simulink model "Model2_V032_R_T4"  (R2023a)
settings: Solver=ode14x  StartTime=0.0  StopTime=Inf  FixedStep=ts  MaxStep=ts  RelTol=1e-5
values from neighbouring files (symbols this model uses):
  ausrollen_a_v = parameters.ausrollen_a_v    [efficiencycalc.m]    (also in parameters_initials.mat = 1)
  bremspunkte = parameters.bremspunkte    [efficiencycalc.m]    (also in parameters_initials.mat = [6100  280  8; 10400  500  3; 14100  550  8; 17729  0  1])
  brennstoffzellen_eta_kennfeld = parameters.brennstoffzellen_eta_kennfeld    [efficiencycalc.m]    (also in parameters_initials.mat = )
  brennstoffzellen_ui_kennfeld = parameters.brennstoffzellen_ui_kennfeld    [efficiencycalc.m]    (also in parameters_initials.mat = )
  coeffs_motor_moment = parameters.coeffs_motor_moment    [efficiencycalc.m]    (also in parameters_initials.mat = [30 30 30 5 7.5 10 0 0 0 6000 6000 6000 ... (30 elements, 3x)
  coeffs_motor_wirkungsgrad = parameters.coeffs_motor_wirkungsgrad    [efficiencycalc.m]    (also in parameters_initials.mat = [30 30 30 5 7.5 10 0 0 0 6000 6000 6000 ... (39 elements, 3x)
  fahrzeug_parameter = parameters.fahrzeug_parameter    [efficiencycalc.m]    (also in parameters_initials.mat = )
  strategie_parameter = parameters.strategie_parameter    [efficiencycalc.m]    (also in parameters_initials.mat = )
  strecke = parameters.strecke    [efficiencycalc.m]    (also in parameters_initials.mat = )
  ts = parameters.ts    [efficiencycalc.m]    (also in parameters_initials.mat = 0.01)
  U_moment = parameters.U_moment    [efficiencycalc.m]    (also in parameters_initials.mat = [30 3])
  U_wirkungsgrad = parameters.U_wirkungsgrad    [efficiencycalc.m]    (also in parameters_initials.mat = [30 3])
  umwelt_parameter = parameters.umwelt_parameter    [efficiencycalc.m]    (also in parameters_initials.mat = )
  zwangsgas = zeros(length(strecke.x),strecke.Rundenzahl)    [Automatisierung_Model_2.m]    (also in efficiencycalc.m; parameters_initials.mat = [0 0 0 0 0 0 0 0 0 0 0 0 ... (2563 elements, 233x11)])
libraries: simulink x1
(part 3 of 3)

== matlab function Model2_V032_R_T4/Motorsteuerung/Kennfeld MC und Motor zusammen/Bestimmung_Wirkungsgrad_aus_Polynomen ==
  data: I input; eta_motor output; U_SC input; n_motor input; eta_U_down output; eta_U_up output; U_wirkungsgrad input; coeffs_motor_wirkungsgrad input; eta_U_down_I_down output; eta_U_down_I_up output; eta_U_up_I_down output; eta_U_up_I_up output
function [eta_motor , eta_U_down , eta_U_up , eta_U_down_I_down , eta_U_down_I_up , eta_U_up_I_down , eta_U_up_I_up ]  = fcn( I , U_SC , n_motor , U_wirkungsgrad , coeffs_motor_wirkungsgrad )
%% Bestimmung Wirkungsgrad aus Polynomen
% Hydro2Motion
% Prototyp: Homer
% Stand: 23.01.2020
% edited: Robin Nedella

%% Eingang
% I:                        [A]     aktuell gefahrener Strom
% U_SC:                     [V]     aktuelle Spannung in den SuperCaps, also aktuelle Spannung am Motorcontroller
% n_motor:                  [rps]   aktuelle Motordrehzahl
% coeffs_motor_wirkungsgrad:[]      Matrix, in welcher die Koeffizienten der Polynome hinterlegt sind (Spalte 1: Strom, 2: Spanung, ab 3: Koeffizienten)
% U_wirkungsgrad:           [V]     Vektor, in welchem die Spannungen stehen, welche in coeffs hinterlegt

%% Ausgang
% eta_motor:                [-]     aktueller Wirkungsgrad Motor bei aktuellem Strom und aktueller Spannung
% eta_U_down:               [-]     aktueller Wirkungsgrad Motor bei nächst kleinerem Strom und aktueller Spannung
% eta_U_up:                 [-]     aktueller Wirkungsgrad Motor bei nächst größerem Strom und aktueller Spannung

%%
n_motor = n_motor * 60; % Polynome basieren auf RPM, nicht RPS

%% Initialisierung
U_down = 0; % nächst kleinere Spannung, für welche Polynome hinterlegt
U_up = 0;   % nächst größere Spannung, für welche Polynome hinterlegt

U_down_I_down = 0; % nächst kleinerer Strom für untere Spannung, für welchen Polynom hinterlegt
U_up_I_down = 0;   % nächst kleinerer Strom für obere Spannung, für welchen Polynom hinterlegt
U_down_I_up = 0;   % nächst größerer Strom für untere Spannung, für welchen Polynom hinterlegt
U_up_I_up = 0;     % nächst größerer Strom für obere Spannung, für welchen Polynom hinterlegt

I_U_down = zeros(1,2);
I_U_up = zeros(1,2);

row_U_down_I_down = 0;  % Zeile, in welcher Koeffizienten für nächst kleineren Strom und nächst kleineren Spannung steht
row_U_down_I_up = 0;    % Zeile, in welcher Koeffizienten für nächst kleineren Strom und nächst größeren Spannung steht
row_U_up_I_down = 0;    % Zeile, in welcher Koeffizienten für nächst größeren Strom und nächst kleineren Spannung steht
row_U_up_I_up = 0;      % Zeile, in welcher Koeffizienten für nächst größeren Strom und nächst größerer Spannung steht

n_motor_U_down_I_down = 0;  % Motordrehzahl, mit welcher das Polynom ausgewertet wird (Gültigkeitsbereich Polynom beachtet) nächst kleinere Spannung und nächst kleinerer Strom
n_motor_U_down_I_up = 0;    % Motordrehzahl, mit welcher das Polynom ausgewertet wird (Gültigkeitsbereich Polynom beachtet) nächst kleinere Spannung und nächst größerer Strom
n_motor_U_up_I_down = 0;    % Motordrehzahl, mit welcher das Polynom ausgewertet wird (Gültigkeitsbereich Polynom beachtet) nächst größere Spannung und nächst kleinerer Strom
n_motor_U_up_I_up = 0;      % Motordrehzahl, mit welcher das Polynom ausgewertet wird (Gültigkeitsbereich Polynom beachtet) nächst größere Spannung und nächst größerer Strom

eta_U_down_I_down = 0;  % aktueller Wirkungsgrad bei nächst kleinerer Spannung und nächst kleinerem Strom
eta_U_down_I_up = 0;    % aktueller Wirkungsgrad bei nächst kleinerer Spannung und nächst größerem Strom
eta_U_up_I_down = 0;    % aktueller Wirkungsgrad bei nächst größerer Spannung und nächst kleinerem Strom
eta_U_up_I_up = 0;      % aktueller Wirkungsgrad bei nächst größerer Spannung und nächst größerem Strom

eta_U_down = 0;         % aktueller Wirkungsgrad bei nächst kleinerer Spannung und aktuellem Strom
eta_U_up = 0;           % aktueller Wirkungsgrad bei nächst größerer Spannung und aktuellem Strom

eta_motor = 1;          % aktueller Wirkungsgrad bei aktuellem Strom und aktueller Spannung (hier: Initialisierung)
%%
if I ~= 0   % wenn gleich null, dann eta_motor = 0 (es muss nichts berechnet werden)
    
    %% suche 2 nächsten Spannungen
        % wenn unter kleinster: nimm kleinste Spannung
    if U_SC < U_wirkungsgrad(1,1)       % wenn aktuelle Spannung kleiner als kleinste im KF hinterlegte
        U_down = U_wirkungsgrad(1,1);       % nächst kleinere Spannung ist kleinste hinterlegte Spannung
        U_up = U_wirkungsgrad(1,1);         % nächst größere Spannung ist kleinste hinterlegte Spannung
        I_U_down = zeros(U_wirkungsgrad(1,2),2);       % Initialisierung des Vektors, wo Ströme, welche bei nächst kleinerer Spannung im Kennfeld hinterlegt sind, gespeichert werden
        I_U_up = zeros(U_wirkungsgrad(1,2),2);         % Initialisierung des Vektors, wo Ströme, welche bei nächst größerer Spannung im Kennfeld hinterlegt sind, gespeichert werden
    elseif U_SC > U_wirkungsgrad(end,1) % wenn aktuelle Spannung größer als größte im KF hinterlegte
        U_down = U_wirkungsgrad(end,1);     % nächst kleinere Spannung ist größte hinterlegte Spannung
        U_up = U_wirkungsgrad(end,1);       % nächst größere Spannung ist größte hinterlegte Spannung
        I_U_down = zeros(U_wirkungsgrad(end,2),2);       % Initialisierung des Vektors, wo Ströme, welche bei nächst kleinerer Spannung im Kennfeld hinterlegt sind, gespeichert werden
        I_U_up = zeros(U_wirkungsgrad(end,2),2);         % Initialisierung des Vektors, wo Ströme, welche bei nächst größerer Spannung im Kennfeld hinterlegt sind, gespeichert werden
    else                                % dann liegt aktuelle Spannung an den Grenzen der m KF hinterlegten Spannungen oder dazwischen
        for j = 1:1:length(U_wirkungsgrad)  % prüfe, ob die gefahrene Spannung direkt im KF hinterlegt ist
           if U_SC == U_wirkungsgrad(j)         % wenn die gefahrene Spannung direkt im KF hinterlegt ist
               U_down = U_SC;                       % dann muss nicht interpoliert werden
               U_up = U_SC;
               I_U_down = zeros(U_wirkungsgrad(j,2),2);       % Initialisierung des Vektors, wo Ströme, welche bei nächst kleinerer Spannung im Kennfeld hinterlegt sind, gespeichert werden
               I_U_up = zeros(U_wirkungsgrad(j,2),2);         % Initialisierung des Vektors, wo Ströme, welche bei nächst größerer Spannung im Kennfeld hinterlegt sind, gespeichert werden
               break;
           elseif U_SC < U_wirkungsgrad(j)      % ansonsten: finde die beiden im Kennfeld hinterlegten Spannungen, zwischen welchen die gefahrene Spannung liegt
               U_down = U_wirkungsgrad(j-1);        % Spannung im Kennfeld, welche am nächsten auf kleineren Seite an die gefahrene Spannung kommt
               U_up = U_wirkungsgrad(j);            % Spannung im Kennfeld, welche am nächsten auf größerer Seite an die gefahrene Spannung kommt
               I_U_down = zeros(U_wirkungsgrad(j-1,2),2);       % Initialisierung des Vektors, wo Ströme, welche bei nächst kleinerer Spannung im Kennfeld hinterlegt sind, gespeichert werden
               I_U_up = zeros(U_wirkungsgrad(j,2),2);         % Initialisierung des Vektors, wo Ströme, welche bei nächst größerer Spannung im Kennfeld hinterlegt sind, gespeichert werden
               break;
           end
        end
    end
    
    %% speichere jeweils die hinterlegten Ströme, 1. Spalte: in welcher Zeile von coeffs_motor_wirkungsgrad steht der Strom; 2. Spalte: Strom
         % für untere Spannung (I_U_down)
    for j = 1:1:length(coeffs_motor_wirkungsgrad(:,1))
        if coeffs_motor_wirkungsgrad(j,1) == U_down
            k = j;
            m = 1;
            while coeffs_motor_wirkungsgrad(k,1) == U_down
                I_U_down(m,2) = coeffs_motor_wirkungsgrad(k,2);
                I_U_down(m,1) = k;
                m = m + 1;
                k = k + 1;
                if k > length(coeffs_motor_wirkungsgrad(:,1))    % dann steht in der nächsten Zeile nicht mehr U_down
                    break;
                end
            end
            break;
        end        
    end
        % für obere Spannung (I_U_up)
    for j = 1:1:length(coeffs_motor_wirkungsgrad(:,1))
        if coeffs_motor_wirkungsgrad(j,1) == U_up
            k = j;
            m = 1;
            while coeffs_motor_wirkungsgrad(k,1) == U_up
                I_U_up(m,2) = coeffs_motor_wirkungsgrad(k,2);   % 2. Spalte: Strom
                I_U_up(m,1) = k;                                % 1. Spalte: Zeile aus coeffs_motor_wirkungsgrad, in welcher der Strom steht
                m = m + 1;
                k = k + 1;
                if k > length(coeffs_motor_wirkungsgrad(:,1))    % dann steht in der nächsten Zeile nicht mehr U_up
                    break;
                end
            end
            break;
        end        
    end
    
    %% suche für untere und obere Spannung jeweils die 2 nächsten Ströme und speichere die Zeile, wo sie in coeffs_motor_wirkungsgrad zu finden sind
        % untere Spannung
    if I < I_U_down(1,2)            % Gültigkeitsbereich beachten! (wenn außerhalb, dann nimm Wert von letztem hinterlegten)
       row_U_down_I_down = I_U_down(1,1);
       row_U_down_I_up = I_U_down(1,1);
       U_down_I_down = I_U_down(1,2);
       U_down_I_up = I_U_down(1,2);
    elseif I > I_U_down(end,2)
       row_U_down_I_down = I_U_down(end,1);
       row_U_down_I_up = I_U_down(end,1);
       U_down_I_down = I_U_down(end,2);
       U_down_I_up = I_U_down(end,2);
    else
        for j = 1:1:length(I_U_down)
          if I == I_U_down(j,2)                 % wenn gefahrene Strom dirket im Kennfeld hinterlegt ist
              row_U_down_I_down = I_U_down(j,1);
              row_U_down_I_up = I_U_down(j,1);
              U_down_I_down = I_U_down(j,2);
              U_down_I_up = I_U_down(j,2);
              break;
          elseif I < I_U_down(j,2)
              row_U_down_I_down = I_U_down(j-1,1);
              row_U_down_I_up = I_U_down(j,1);
              U_down_I_down = I_U_down(j-1,2);
              U_down_I_up = I_U_down(j,2);
              break;
          end
        end
    end
        % obere Spannung
    if I < I_U_up(1,2)
       row_U_up_I_down = I_U_up(1,1);
       row_U_up_I_up = I_U_up(1,1);
       U_up_I_down = I_U_up(1,2);
       U_up_I_up = I_U_up(1,2);
    elseif I > I_U_up(end,2)
       row_U_up_I_down = I_U_up(end,1);
       row_U_up_I_up = I_U_up(end,1);
       U_up_I_down = I_U_up(end,2);
       U_up_I_up = I_U_up(end,2);
    else
        for j = 1:1:length(I_U_up)
          if I == I_U_up(j,2)                 % wenn gefahrene Strom dirket im Kennfeld hinterlegt ist
              row_U_up_I_down = I_U_up(j,1);
              row_U_up_I_up = I_U_up(j,1);
              U_up_I_down = I_U_up(j,2);
              U_up_I_up = I_U_up(j,2);
              break;
          elseif I < I_U_up(j,2)
              row_U_up_I_down = I_U_up(j-1,1);
              row_U_up_I_up = I_U_up(j,1);
              U_up_I_down = I_U_up(j-1,2);
              U_up_I_up = I_U_up(j,2);
              break;
          end
        end
    end
    
    %% Gültigkeitsbereich Polynome beachten
        % Motordrehzahl, mit welcher Polynom für nächst kleinere Spannung und nächst kleinerem Strom ausgewertet wird
    if n_motor < coeffs_motor_wirkungsgrad(row_U_down_I_down,3)
        n_motor_U_down_I_down = coeffs_motor_wirkungsgrad(row_U_down_I_down,3);
    elseif n_motor > coeffs_motor_wirkungsgrad(row_U_down_I_down,4)
        n_motor_U_down_I_down = coeffs_motor_wirkungsgrad(row_U_down_I_down,4);
    else
        n_motor_U_down_I_down = n_motor;
    end
        % Motordrehzahl, mit welcher Polynom für nächst kleinere Spannung und nächst größerem Strom ausgewertet wird
    if n_motor < coeffs_motor_wirkungsgrad(row_U_down_I_up,3)
        n_motor_U_down_I_up = coeffs_motor_wirkungsgrad(row_U_down_I_up,3);
    elseif n_motor > coeffs_motor_wirkungsgrad(row_U_down_I_up,4)
        n_motor_U_down_I_up = coeffs_motor_wirkungsgrad(row_U_down_I_up,4);
    else
        n_motor_U_down_I_up = n_motor;
    end
        % Motordrehzahl, mit welcher Polynom für nächst größere Spannung und nächst kleinerem Strom ausgewertet wird
    if n_motor < coeffs_motor_wirkungsgrad(row_U_up_I_down,3)
        n_motor_U_up_I_down = coeffs_motor_wirkungsgrad(row_U_up_I_down,3);
    elseif n_motor > coeffs_motor_wirkungsgrad(row_U_up_I_down,4)
        n_motor_U_up_I_down = coeffs_motor_wirkungsgrad(row_U_up_I_down,4);
    else
        n_motor_U_up_I_down = n_motor;
    end
            % Motordrehzahl, mit welcher Polynom für nächst größere Spannung und nächst größerem Strom ausgewertet wird
    if n_motor < coeffs_motor_wirkungsgrad(row_U_up_I_up,3)
        n_motor_U_up_I_up = coeffs_motor_wirkungsgrad(row_U_up_I_up,3);
    elseif n_motor > coeffs_motor_wirkungsgrad(row_U_up_I_up,4)
        n_motor_U_up_I_up = coeffs_motor_wirkungsgrad(row_U_up_I_up,4);
    else
        n_motor_U_up_I_up = n_motor;
    end
    
    %% Werte (Wirkungsgrad / Moment) aus Polynom berechnen
        % aktueller Wirkungsgrad für nächst kleineren Strom bei nächst kleinerer Spannung
    eta_U_down_I_down = polyval( fliplr( coeffs_motor_wirkungsgrad( row_U_down_I_down , 5:end )) , n_motor_U_down_I_down);
        % aktueller Wirkungsgrad für nächst größeren Strom bei nächst kleinerer Spannung
    eta_U_down_I_up   = polyval( fliplr( coeffs_motor_wirkungsgrad( row_U_down_I_up   , 5:end )) , n_motor_U_down_I_up);
        % aktueller Wirkungsgrad für nächst kleineren Strom bei nächst größerer Spannung
    eta_U_up_I_down   = polyval( fliplr( coeffs_motor_wirkungsgrad( row_U_up_I_down   , 5:end )) , n_motor_U_up_I_down);
        % aktueller Wirkungsgrad für nächst kleineren Strom bei nächst kleinerer Spannung
    eta_U_up_I_up     = polyval( fliplr( coeffs_motor_wirkungsgrad( row_U_up_I_up     , 5:end )) , n_motor_U_up_I_up);
        
    %% Interpoliere jeweils zwischen den Strömen linear
        % interpolierter Wirkungsgrad des aktuellen Stroms bei nächst kleinerer Spannung
    if U_down_I_down == U_down_I_up         % dann muss nicht interpoliert werden
        eta_U_down = eta_U_down_I_down;         % nimm eta_U_down_I_down oder eta_U_down_I_up
    else                                    % dann muss interpoliert werden
        eta_U_down = (I - U_down_I_down) * (eta_U_down_I_up - eta_U_down_I_down) / (U_down_I_up - U_down_I_down) + eta_U_down_I_down;
    end
        % interpoliere Wirkungsgrad des aktuellen Stroms bei nächst größerer Spannung
    if U_up_I_down == U_up_I_up             % dann muss nicht interpoliert werden
        eta_U_up = eta_U_up_I_down;             % nimm eta_U_up_I_down oder eta_U_up_I_up
    else                                    % dann muss interpoliert werden
        eta_U_up   = (I - U_up_I_down)   * (eta_U_up_I_up   - eta_U_up_I_down)   / (U_up_I_up   - U_up_I_down)   + eta_U_up_I_down;
    end
    
    %% Interpoliere zwischen den Spannungen dann linear
        % wenn udown = uup dann keine interpolation nötig
    if U_down == U_up                       % dann muss nicht interpoliert werden
        eta_motor = eta_U_down;                 % nimm eta_U_down oder eta_U_up
    else
        eta_motor = (U_SC - U_down) * (eta_U_up - eta_U_down) / (U_up - U_down) + eta_U_down;
    end

end

end

== matlab function Model2_V032_R_T4/Motorsteuerung/Kennfeld MC und Motor zusammen/for testing: if constant offset of Motor Efficiency ==
  data: eta_normal input; eta_real output; delta_eta input
function eta_real = fcn(eta_normal , delta_eta)

if eta_normal == 1
    eta_real = eta_normal;
else
    eta_real = eta_normal + delta_eta;
end

end

== matlab function Model2_V032_R_T4/Fahrer // Strategie/aktuelle Streckendaten einlesen ==
  data: steigung_aktuell output; position input; position_runde output; fertige_runden output; distanz_3d input; distanz_2d input; steigung input; hoehe input; hoehe_aktuell output; radius input; radius_aktuell output; hoehenradius input; hoehenradius_aktuell output; wegpunkt output
function [ steigung_aktuell , position_runde , fertige_runden , hoehe_aktuell , radius_aktuell , hoehenradius_aktuell , wegpunkt ] = fcn( position , distanz_3d , distanz_2d , steigung , hoehe , radius , hoehenradius )
%% aktuelle Streckendaten einlesen
% Hydro2Motion
% Prototyp: Homer
% Stand: 23.01.2020
% edited: Robin Nedella

%% Eingang
% position:             [m]     insgesamt bereits zurückgelegter Weg seit Start der Simulation
% distanz_3d:           [-]     Vektor aus strecke-Struct, in welchem Distanz im Raum zwischen Wegpunkten aufaddiert steht
% distanz_2d:           [-]     Vektor aus strecke-Struct, in welchem Distanz in 2D (Draufsicht auf die Strecke) zwischen Wegpunkten aufaddiert steht
% steigung:             [-]     Vektor aus strecke-Struct, in welchem die Steigung in [rad] je Wegpunkt steht
% hoehe:                [-]     Vektor aus strecke-Struct, in welchem die Höhe [m] je Wegpunkt steht
% radius:               [-]     Vektor aus strecke-Struct, in welchem der Kurvenradius [m] je Wegpunkt steht
% hoehenradius:         [-]     Vektor aus strecke-Struct, in welchem der Höhenradius [m] je Wegpunkt steht

%% Ausgang
% steigung_aktuell:     [rad]   in der aktuellen Position der Runde vorliegende Steigung [rad], linear interpoliert aus benachbarten bekannten Steigungen in "steigung" aus strecke-Struct
% position_runde:       [m]     in der aktuellen Runde zurückgelegter Weg
% fertige_runden:       [-]     seit Start der Simulation bereits absolvierte Rundenzahl
% hoehe_aktuell:        [m]     in der aktuellen Position der Runde vorliegende Höhe [m], linear interpoliert aus benachbarten bekannten Höhen in "hoehe" aus strecke-Struct
% radius_aktuell:       [m]     in der aktuellen Position der Runde vorliegender Kurvenradius [m], linear interpoliert aus benachbarten bekannten Kurvenradien in "radius" aus strecke-Struct
% hoehenradius_aktuell: [m]     in der aktuellen Position der Runde vorliegender Höhenradius [m], linear interpoliert aus benachbarten bekannten Höhenradien in "hoehenradius" aus strecke-Struct
% wegpunkt:             [-]     Zeilennummer des letzten Wegpunktes aus dem strecke-Struct, welcher zuletzt passiert wurde

%% Berechnung

%% Anzahl der bereits absolvierten Runden und Position in aktueller Runde
rundenlaenge   = distanz_3d(end);                            % [m] Länge einer Runde (distanz_3d)
fertige_runden = fix(position / rundenlaenge);               % [-] Anzahl der bereits absolvierten Runden ("fix" rundet ab)
position_runde = position - fertige_runden * rundenlaenge;   % [m] Position in der aktuellen Runde

% Zeilen bestimmen, zwischen denen interpoliert werden soll
i = 2;      % Initialisierung
while (position_runde > distanz_3d(i))
    i = i + 1;
end
wegpunkt = i;                               % "i" ist die Zeile des letzten Wegpunktes aus der mat, welcher bereits passiert wurde

% Bestimmung der aktuellen Steigung
steigung_aktuell =  (steigung(i) - steigung(i-1)) / (distanz_3d(i) - distanz_3d(i-1)) * (position_runde - distanz_3d(i-1)) + steigung(i-1); 

% Bestimmung der aktuellen Höhe
hoehe_aktuell = (hoehe(i) - hoehe(i-1)) / (distanz_3d(i) - distanz_3d(i-1)) * (position_runde - distanz_3d(i-1)) + hoehe(i-1);

% Bestimmung des aktuellen Kurvenradius
radius_aktuell =  (radius(i) - radius(i-1)) / (distanz_3d(i) - distanz_3d(i-1)) * (position_runde - distanz_3d(i-1)) + radius(i-1);

% Bestimmung des aktuellen Höhenradius
hoehenradius_aktuell =  (hoehenradius(i) - hoehenradius(i-1)) / (distanz_2d(i) - distanz_2d(i-1)) * (position_runde - distanz_2d(i-1)) + hoehenradius(i-1);

end

== matlab function Model2_V032_R_T4/Fahrer // Strategie/Strategie_Fahrer ==
  data: fps_last input; fps_neu output; v input; v_durch input; dv_min input; dv_max input; i_getriebe_vec input; i_getriebe output; radius input; Gas_Kurve input; crit_radius_gas input; v_low input; dv_low_down input; dv_low_up input; wegpunkt input; cuts input; track_length input
function [ fps_neu , i_getriebe ]    = fcn( fps_last , v , v_durch , dv_min , dv_max , i_getriebe_vec , radius , Gas_Kurve, crit_radius_gas , v_low , dv_low_down , dv_low_up , wegpunkt , cuts, track_length)
%% Strategie Fahrer
% Hydro2Motion
% Prototyp: Homer
% Stand: 23.01.2020
% edited: Robin Nedella

%% Eingang
% fps_last:             [-]     aktuelle Fahrpedalstellung (0: kein Gas, 1: Gas)
% v:                    [m/s]   aktuelle Geschwindigkeit
% v_durch:              [m/s]   Durchschnittsgeschwindigkeit bestimmt aus vorgeg. Gesamtzeit und Gesamtstrecke
% dv_min:               [m/s]   untere Differenz zur Durchschnittsgeschwindigkeit. Wenn diese unterschritten wird, wird Gas gegeben (fps=1)
% dv_max:               [m/s]   obere Differenz zur Durchschnittsgeschwindigkeit. Wenn diese überschritten wird, wird kein Gas mehr gegeben (fps=0)
% i_getriebe_vec:       [-]     Vektor mit möglichen Übersetzungen
% radius:               [m]     aktuell vorliegender Kurvenradius
% Gas_Kurve:            [-]     Ergebnis aus "Kurvenüberwachung" (0: kein Gas wegen Kurve, 1: Gas geben ist ok)
% crit_radius_gas:      [m]     kritischer Kurvenradius, ab dessen Unterschreiten kein Gas gegeben werden darf (da ineffizient, wenn in Kurve Gas gegeben wird!)
% v_low:                [m/s]   Mindestgeschwindigkeit. Wenn unterschritten --> Gas geben, auch wenn Kurve
% dv_low_down:          [m/s]   untere Differenz zur Mindestgeschwindigkeit. 
% dv_low_up:            [m/s]   obere Differenz zur Mindestgeschwindigkeit.
%% Addition of wegpunkt and cuts
% track_length          [-]     Length of wegpunkt(track data)
% wegpunkt:             [-]     Point of the road
% cuts:                 [-]     Point of the road
%% Ausgang
% fps_neu:              [-]     neu vorgegebene Fahrpedalstellung (0: kein Gas, 1: Gas)
% i_getriebe:           [-]     gewählte Übersetzung

%% Aktuelle Strategie

fps_neu = 0;        % Initialisierung

i=1;
if wegpunkt >= 0 && wegpunkt <= cuts(1)
    i = 1;
elseif wegpunkt > cuts(1) && wegpunkt <= cuts(2)
    i = 2;
elseif wegpunkt > cuts(2) && wegpunkt <= cuts(3)
    i = 3;
elseif wegpunkt > cuts(3) && wegpunkt <= cuts(4)
    i = 4;
elseif wegpunkt > cuts(4) && wegpunkt <= cuts(5)
    i = 5;
elseif wegpunkt > cuts(5) && wegpunkt <= cuts(6)
    i = 6;
elseif wegpunkt > cuts(6) && wegpunkt <= cuts(7)
    i = 7;
elseif wegpunkt > cuts(7) && wegpunkt <= length(track_length)
    i = 8;
end

% anhand v_durch und Bandbreite mit max. Abweichung zur v_durch (+/-) wird bei Überschreiten durch fps_neu nachgeregelt
v_min = v_durch + dv_min(i);    % untere Grenze der Bandbreite
v_max = v_durch + dv_max(i);    % obere Grenze der Bandbreite

if fps_last == 0 && v < v_min                        % Unterschreiten der unteren Grenze während Ausrollen
    fps_neu = 1;
elseif fps_last == 1 && v > v_max                    % Überschreiten der oberen Grenze während Gasgeben
    fps_neu = 0;
elseif fps_last == 1 && v > v_min && v < v_max       % weiter Gasgeben, wenn zwischen Grenzen und Beschleunigen
    fps_neu = 1;
elseif fps_last == 1 && v < v_min                    % falls das unmögliche möglich wird... (so hohe Widerstände, dass so schnell abgebremst wird, dass kein Berechnungsschritt zwischen oberer und unterer Grenze)
    fps_neu = 1;
end

% Kein Gas, wenn Kurvenradius kleiner crit_radius_gas (da in der Kurve nicht Gas gegeben werden soll)
if radius < crit_radius_gas
    fps_neu = 0;
end

% Vorausrechnen, ob nächsten ... Sekunden Kurve kommt (in "Kurvenüberwachung: "Gas_Kurve")
if Gas_Kurve == 0   
    fps_neu = 0;                               % kein Gas, falls Kurve zu nah und Gefahr läuft, auch in der Kurve noch Gas zu geben
end

%% Minimale Geschwindigkeit
% Wenn minimale Geschwindigkeit unterschritten, trotzdem Gas geben! und dies nicht nur punktuell, bis v_low überschritten, sondern bis v_low_up erreicht, dann Ausrollen bis v_low erreicht!
% !!! dies soll jedoch nicht das oben stehende überstimmen, sondern ledigleich in Kraft treten, wenn nach der oben stehenden Logik KEIN GAS gegeben wird! 
if fps_neu == 0
    % anhand v_low und Bandbreite mit max. Abweichung zur v_low (+/-) wird bei Überschreiten durch Gas_Kurve_neu nachgeregelt
    v_low_down = v_low - dv_low_down;    % untere Grenze der Bandbreite
    v_low_up   = v_low + dv_low_up;      % obere Grenze der Bandbreite

    if fps_last == 0 && v < v_low_down                        % Unterschreiten der unteren Grenze während Ausrollen
        fps_neu = 1;
    elseif fps_last == 1 && v > v_low_up                      % Überschreiten der oberen Grenze während Gasgeben
        fps_neu = 0;
    elseif fps_last == 1 && v > v_low_down && v < v_low_up    % weiter Gasgeben, wenn zwischen Grenzen und Beschleunigen
        fps_neu = 1;
    elseif fps_last == 1 && v < v_low_down                    % falls das unmögliche möglich wird... (so hohe Widerstände, dass so schnell abgebremst wird, dass kein Berechnungsschritt zwischen oberer und unterer Grenze)
        fps_neu = 1;
    end
end

%% Berechnung i_getriebe
i_getriebe = i_getriebe_vec(1);                % aktuell nur 1 Gang implementiert

end

== matlab function Model2_V032_R_T4/Energieversorgung/Berechnung delta Spannung Entladung Motor ==
  data: I input; delta_U_SC_discharge_Motor output; C_SC input; ts input; t input
function delta_U_SC_discharge_Motor = fcn( I , C_SC , ts , t )
%% Berechnung Entladung durch Motor
% Hydro2Motion
% Prototyp: Homer
% Stand: 23.01.2020
% edited: Timo Freilinger

%% Eingang
% I:                     [A]    aktuell von Motorcontroller benötigter Strom
% C_SC:                  [F]    Kapazität der Kondensatoren
% ts:                    [sec]  Zeitschritt der Berechnung
% t:                     [sec]  aktuelle Simulationszeit

%% Ausgang
% delta_U_SC_discharge:  [V]    Betrag der Spannung, um welchen die SC aktuell entladen werden

%% Berechnung

if t == 0                                    % initial zu Beginn der Simulation
    delta_U_SC_discharge_Motor = 0;                % werden die SC nicht entladen
elseif I == 0                                % wenn kein Strom entnommen wird
    delta_U_SC_discharge_Motor = 0;                % werden die SC nicht entladen
else                                         % ansonsten werden die SC entladen
    delta_U_SC_discharge_Motor = - I * ts / C_SC;  % Spannungsabfall der SC im Simulationsschritt ts
end

end

== matlab function Model2_V032_R_T4/Fahr-Dynamik/Widerstände über Ausrollkurven/MATLAB Function ==
  data: v input; F_W_ausrollkurven output; ausrollen_a_v input
function F_W_ausrollkurven = fcn(v,ausrollen_a_v)

F_W_ausrollkurven = polyval(ausrollen_a_v,v);

end
